simulink model "overall_simulator"  (R2017a)
settings: Solver=VariableStepAuto  StartTime=0.0  StopTime=100  RelTol=1e-3
InitFcn:
  | Iyy_lbft2= 261.096376; %last updated 7 Dec 2018
  | Iyy = 0.04214011 *Iyy_lbft2;
libraries: simulink x5, aerolibconvert2 x4, shared3dof x1, aerolibasang x1
settings Model: Creator=Devansh  LastModifiedBy=Devansh

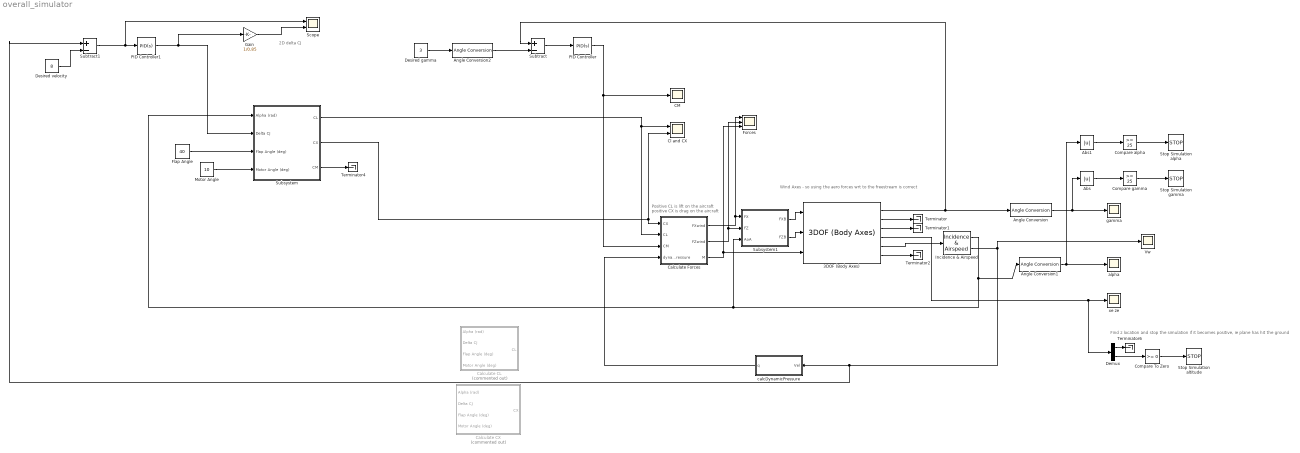
== system overall_simulator ==
  note: 2D delta CJ
  note: Positive CL is lift on the aircraft
      | positive CX is drag on the aircraft
  note: Find z location and stop the simulation if it becomes positive, ie plane has hit the ground
  note: Wind Axes - so using the aero forces wrt to the freestream is correct
  3DOF (Body Axes) : shared3dof/3DOF (Body Axes)  units=Metric (MKS)  mtype=Fixed  v_ini=5  theta_ini=-5*pi/180  alpha_ini=12*pi/180  q_ini=0  pos_ini=[0 -100]  mass=20  mass_e=0.5  mass_f=3.0  Iyy=Iyy  Iyy_e=0.5  Iyy_f=3.0  g_in=Internal  g=9.81  vre_flag=on  abi_flag=off
  Abs : Abs
  Abs1 : Abs
  Angle Conversion : aerolibconvert2/Angle Conversion  IU=rad  OU=deg
  Angle Conversion1 : aerolibconvert2/Angle Conversion  IU=rad  OU=deg
  Angle Conversion2 : aerolibconvert2/Angle Conversion  IU=deg  OU=rad
  CM : Scope
  Calculate CL : Subsystem  Commented=on
  Calculate CX : Subsystem  Commented=on
  Calculate Forces : Subsystem
  Cl and CX : Scope  NumInputPorts=2
  Compare To Zero : simulink/Logic and Bit Operations/Compare To Zero  relop=>=  OutDataTypeStr=boolean
  Compare alpha : simulink/Logic and Bit Operations/Compare To Constant  relop=>=  const=25  OutDataTypeStr=boolean
  Compare gamma : simulink/Logic and Bit Operations/Compare To Constant  relop=>=  const=25  OutDataTypeStr=boolean
  Demux : Demux  Outputs=2
  "Desired gamma " : Constant  Value=3
  Desired velocity : Constant  Value=8
  Flap Angle : Constant  Value=40
  Forces : Scope  NumInputPorts=3
  Gain : Gain  Gain=1/0.85
  Incidence & Airspeed : aerolibasang/Incidence  & Airspeed
      settings: SourceProductName=Aerospace Blockset  SourceProductBaseCode=AE
  Motor Angle : Constant  Value=10
  PID Controller : simulink/Continuous/PID Controller  Controller=PID  TimeDomain=Continuous-time  SampleTime=-1  IntegratorMethod=Forward Euler  FilterMethod=Forward Euler  Form=Parallel  UseFilter=on  ControllerParametersSource=internal  P=-0.01  I=0  D=-0.05  N=100  InitialConditionSource=internal  InitialConditionForIntegrator=0  InitialConditionForFilter=0  ExternalReset=none  LimitOutput=off  UpperSaturationLimit=0.1  LowerSaturationLimit=-0.1  LinearizeAsGain=off  AntiWindupMode=none  Kb=1  TrackingMode=off  Kt=1  PParamMin=[]  PParamMax=[]  IParamMin=[]  IParamMax=[]  DParamMin=[]  DParamMax=[]  NParamMin=[]  NParamMax=[]  KbParamMin=[]  KbParamMax=[]  KtParamMin=[]  KtParamMax=[]  POutMin=[]  POutMax=[]  IOutMin=[]  IOutMax=[]  DOutMin=[]  DOutMax=[]  NOutMin=[]  NOutMax=[]  KbOutMin=[]  KbOutMax=[]  KtOutMin=[]  KtOutMax=[]  IntegratorOutMin=[]  IntegratorOutMax=[]  FilterOutMin=[]  FilterOutMax=[]  SumOutMin=[]  SumOutMax=[]  SumI1OutMin=[]  SumI1OutMax=[]  SumI2OutMin=[]  SumI2OutMax=[]  SumI3OutMin=[]  SumI3OutMax=[]  SumDOutMin=[]  SumDOutMax=[]  SaturationOutMin=[]  SaturationOutMax=[]  IntegratorContinuousStateAttributes=''  IntegratorStateMustResolveToSignalObject=off  IntegratorRTWStateStorageClass=Auto  FilterContinuousStateAttributes=''  FilterStateMustResolveToSignalObject=off  FilterRTWStateStorageClass=Auto  DifferentiatorICPrevScaledInput=0  DifferentiatorOutMin=[]  DifferentiatorOutMax=[]  InitialConditionSetting=State (most efficient)
  PID Controller1 : simulink/Continuous/PID Controller  Controller=PID  TimeDomain=Continuous-time  SampleTime=-1  IntegratorMethod=Forward Euler  FilterMethod=Forward Euler  Form=Parallel  UseFilter=on  ControllerParametersSource=internal  P=-0.5  I=-2  D=0  N=100  InitialConditionSource=internal  InitialConditionForIntegrator=0  InitialConditionForFilter=0  ExternalReset=none  LimitOutput=on  UpperSaturationLimit=5  LowerSaturationLimit=0  LinearizeAsGain=off  AntiWindupMode=none  Kb=1  TrackingMode=off  Kt=1  PParamMin=[]  PParamMax=[]  IParamMin=[]  IParamMax=[]  DParamMin=[]  DParamMax=[]  NParamMin=[]  NParamMax=[]  KbParamMin=[]  KbParamMax=[]  KtParamMin=[]  KtParamMax=[]  POutMin=[]  POutMax=[]  IOutMin=[]  IOutMax=[]  DOutMin=[]  DOutMax=[]  NOutMin=[]  NOutMax=[]  KbOutMin=[]  KbOutMax=[]  KtOutMin=[]  KtOutMax=[]  IntegratorOutMin=[]  IntegratorOutMax=[]  FilterOutMin=[]  FilterOutMax=[]  SumOutMin=[]  SumOutMax=[]  SumI1OutMin=[]  SumI1OutMax=[]  SumI2OutMin=[]  SumI2OutMax=[]  SumI3OutMin=[]  SumI3OutMax=[]  SumDOutMin=[]  SumDOutMax=[]  SaturationOutMin=[]  SaturationOutMax=[]  IntegratorContinuousStateAttributes=''  IntegratorStateMustResolveToSignalObject=off  IntegratorRTWStateStorageClass=Auto  FilterContinuousStateAttributes=''  FilterStateMustResolveToSignalObject=off  FilterRTWStateStorageClass=Auto  DifferentiatorICPrevScaledInput=0  DifferentiatorOutMin=[]  DifferentiatorOutMax=[]  InitialConditionSetting=State (most efficient)
  Scope : Scope  NumInputPorts=2
  Stop Simulation alpha : Stop
  Stop Simulation altitude : Stop
  Stop Simulation gamma : Stop
  Subsystem : Subsystem
  Subsystem1 : Subsystem
  Subtract : Sum  Inputs=+|-
  Subtract1 : Sum  Inputs=+|-
  Terminator{,1..2,4,6} (5 alike) : Terminator
  Vw : Scope
  alpha : Scope
  calcDynamicPressure : Subsystem  TreatAsAtomicUnit=on
  gamma : Scope
  xe ze : Scope
  wires:
  3DOF (Body Axes)/4 -> xe ze/1, Demux/1
  Angle Conversion/1 -> Abs/1, gamma/1
  Angle Conversion1/1 -> alpha/1, Abs1/1
  Demux/2 -> Compare To Zero/1
  Compare To Zero/1 -> Stop Simulation altitude/1
  Incidence & Airspeed/2 -> Subtract1/1, calcDynamicPressure/1(Vel), Vw/1
  "Desired gamma "/1 -> Angle Conversion2/1
  Subtract/1 -> PID Controller/1
  Angle Conversion2/1 -> Subtract/2
  Subsystem/1(CL) -> Calculate Forces/2(CL), Cl and CX/1
  calcDynamicPressure/1(q) -> Calculate Forces/4(dynamicPressure)
  Calculate Forces/1(FXwind) -> Forces/1, Subsystem1/1(FX)
  Calculate Forces/2(FZwind) -> Forces/2, Subsystem1/2(FZ)
  Calculate Forces/3(M) -> 3DOF (Body Axes)/3, Forces/3
  3DOF (Body Axes)/2 -> Terminator/1
  3DOF (Body Axes)/3 -> Terminator1/1
  3DOF (Body Axes)/6 -> Terminator2/1
  Flap Angle/1 -> Subsystem/3(Flap Angle (deg))
  Subsystem/2(CX) -> Cl and CX/2, Calculate Forces/1(CX)
  Motor Angle/1 -> Subsystem/4(Motor Angle (deg))
  PID Controller1/1 -> Gain/1, Subsystem/2(Delta CJ)
  Compare gamma/1 -> Stop Simulation gamma/1
  Abs/1 -> Compare gamma/1
  Abs1/1 -> Compare alpha/1
  Incidence & Airspeed/1 -> Subsystem1/3(AoA), Subsystem/1(Alpha (rad)), Angle Conversion1/1
  Compare alpha/1 -> Stop Simulation alpha/1
  PID Controller/1 -> Calculate Forces/3(CM), CM/1
  Subsystem/3(CM) -> Terminator4/1
  Demux/1 -> Terminator6/1
  Subtract1/1 -> Scope/1, PID Controller1/1
  Desired velocity/1 -> Subtract1/2
  Gain/1 -> Scope/2
  3DOF (Body Axes)/5 -> Incidence & Airspeed/1
  Subsystem1/1(FXB) -> 3DOF (Body Axes)/1
  Subsystem1/2(FZB) -> 3DOF (Body Axes)/2
  3DOF (Body Axes)/1 -> Subtract/1, Angle Conversion/1

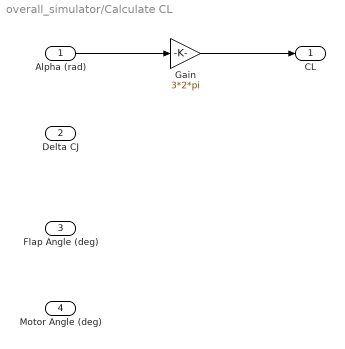
== system overall_simulator/Calculate CL ==
  Alpha (rad) : Inport
  Delta CJ : Inport  Port=2
  Flap Angle (deg) : Inport  Port=3
  Motor Angle (deg) : Inport  Port=4
  Gain : Gain  Gain=3*2*pi
  CL : Outport
  wires:
  Alpha (rad)/1 -> Gain/1
  Gain/1 -> CL/1

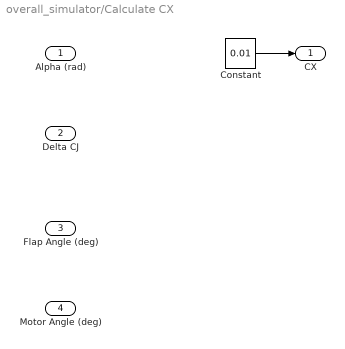
== system overall_simulator/Calculate CX ==
  Alpha (rad) : Inport
  Delta CJ : Inport  Port=2
  Flap Angle (deg) : Inport  Port=3
  Motor Angle (deg) : Inport  Port=4
  Constant : Constant  Value=0.01
  CX : Outport
  wires:
  Constant/1 -> CX/1

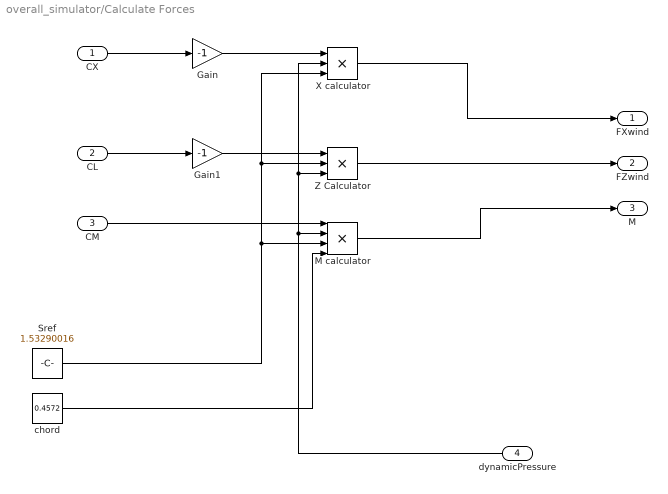
== system overall_simulator/Calculate Forces ==
  CX : Inport
  CL : Inport  Port=2
  CM : Inport  Port=3
  dynamicPressure : Inport  Port=4
  Gain : Gain  Gain=-1
  Gain1 : Gain  Gain=-1
  M calculator : Product  Inputs=4
  Sref : Constant  Value=1.53290016
  X calculator : Product  Inputs=3
  Z Calculator : Product  Inputs=3
  chord : Constant  Value=0.4572
  FXwind : Outport
  FZwind : Outport  Port=2
  M : Outport  Port=3
  wires:
  CM/1 -> M calculator/1
  M calculator/1 -> M/1
  chord/1 -> M calculator/4
  Sref/1 -> X calculator/3, Z Calculator/2, M calculator/3
  X calculator/1 -> FXwind/1
  dynamicPressure/1 -> X calculator/2, Z Calculator/3, M calculator/2
  Z Calculator/1 -> FZwind/1
  CX/1 -> Gain/1
  CL/1 -> Gain1/1
  Gain/1 -> X calculator/1
  Gain1/1 -> Z Calculator/1

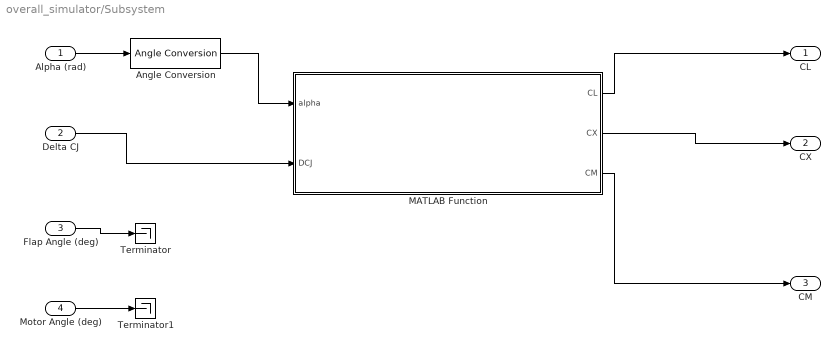
== system overall_simulator/Subsystem ==
  Alpha (rad) : Inport
  Delta CJ : Inport  Port=2
  Flap Angle (deg) : Inport  Port=3
  Motor Angle (deg) : Inport  Port=4
  Angle Conversion : aerolibconvert2/Angle Conversion  IU=rad  OU=deg
  MATLAB Function : MATLAB Function  TreatAsAtomicUnit=on
  Terminator : Terminator
  Terminator1 : Terminator
  CL : Outport
  CX : Outport  Port=2
  CM : Outport  Port=3
  wires:
  Delta CJ/1 -> MATLAB Function/2(DCJ)
  MATLAB Function/1(CL) -> CL/1
  MATLAB Function/2(CX) -> CX/1
  MATLAB Function/3(CM) -> CM/1
  Alpha (rad)/1 -> Angle Conversion/1
  Angle Conversion/1 -> MATLAB Function/1(alpha)
  Flap Angle (deg)/1 -> Terminator/1
  Motor Angle (deg)/1 -> Terminator1/1

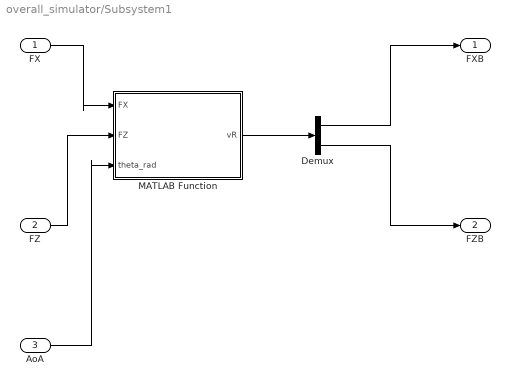
== system overall_simulator/Subsystem1 ==
  FX : Inport
  FZ : Inport  Port=2
  AoA : Inport  Port=3
  Demux : Demux  Outputs=2
  MATLAB Function : MATLAB Function  TreatAsAtomicUnit=on
  FXB : Outport
  FZB : Outport  Port=2
  wires:
  FX/1 -> MATLAB Function/1(FX)
  FZ/1 -> MATLAB Function/2(FZ)
  AoA/1 -> MATLAB Function/3(theta_rad)
  MATLAB Function/1(vR) -> Demux/1
  Demux/1 -> FXB/1
  Demux/2 -> FZB/1

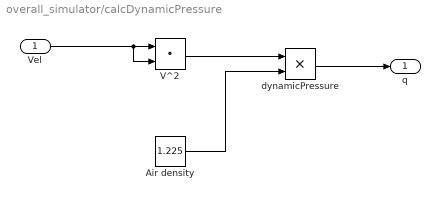
== system overall_simulator/calcDynamicPressure ==
  Vel : Inport
  Air density : Constant  Value=1.225
  V^2 : DotProduct  InputSameDT=on  OutDataTypeStr=Inherit: Inherit via internal rule
  dynamicPressure : Product
  q : Outport
  wires:
  V^2/1 -> dynamicPressure/1
  Air density/1 -> dynamicPressure/2
  Vel/1 -> V^2/2, V^2/1
  dynamicPressure/1 -> q/1

== matlab function overall_simulator/Subsystem1/MATLAB Function ==
  data: FX input; vR output; FZ input; theta_rad input
function vR = rotation(FX, FZ, theta_rad)

v = [FX; FZ];

 R = [cos(theta_rad) -sin(theta_rad); sin(theta_rad) cos(theta_rad)];
 
 vR = R*v;

== matlab function overall_simulator/Subsystem/MATLAB Function ==
  data: alpha input; CL output; DCJ input; CX output; CM output
function [CL,CX,CM] = getCLCXCM_for_df40(alpha, DCJ)

%% convert 3D Delta CJ to 2D

delta_cj=DCJ/0.85;

%% get coefficient matrix
%assumes delta f = 40;
deltaf = 40;

CL_coeffs =[1.34084802984238,0.0922989525732600,-0.000100934251419516,0,0;...
    0.840192956938716,0.0440183793695609,-2.84422877175519e-05,0,0];

CD_coeffs =[0.217559985374938,-0.0212488590862297,0.00119201327474585,0,0;...
    -0.717426345875555,0.0291623276576992,-9.19585265352026e-05,0,0];

CM_coeffs = [-0.209467748915995,0.000759426537477041,-1.11246051270488e-06,0,0;...
    -0.0980528447065869,-0.000645846214599032,7.76293222113931e-06,0,0];

%% get regression results

%get cl
X=[];
for i=0:size(CL_coeffs,1)-1
    X=[X (delta_cj.^i)];
end

cl=X*CL_coeffs(:,1)+alpha.*(X*CL_coeffs(:,2))+alpha.^3.*(X*CL_coeffs(:,3))+deltaf.*(X*CL_coeffs(:,4))+deltaf.^3.*(X*CL_coeffs(:,5));

%get cx
X=[];
for i=0:size(CD_coeffs,1)-1
    X=[X (delta_cj.^i)];
end
cx=X*CD_coeffs(:,1)+alpha.*(X*CD_coeffs(:,2))+alpha.^2.*(X*CD_coeffs(:,3))+deltaf.*(X*CD_coeffs(:,4))+deltaf.^2.*(X*CD_coeffs(:,5));

%get cm
X=[];
for i=0:size(CM_coeffs,1)-1
    X=[X (delta_cj.^i)];
end
cm=X*CM_coeffs(:,1)+alpha.*(X*CM_coeffs(:,2))+alpha.^3.*(X*CM_coeffs(:,3))+deltaf.*(X*CM_coeffs(:,4))+deltaf.^3.*(X*CM_coeffs(:,5));


%% convert to 3D params
AR = 7.5;

e=0.9;
CT=DCJ-1;
CDp=0.05; %profile drag of the rest of the aircraft

CL=0.9*cl;
CX=0.9*cx+CDp+CL.^2./(pi*AR*e+2*CT);
CM = cm;


end
